simulink model "lab2_part1"  (R2023b)
settings: Solver=VariableStepAuto  StartTime=0.0  StopTime=30.0  RelTol=1e-10  AbsTol=1e-10
undefined symbols (not defined in the file): A, B, K
settings Model: Creator=markzhuang  LastModifiedBy=markzhuang

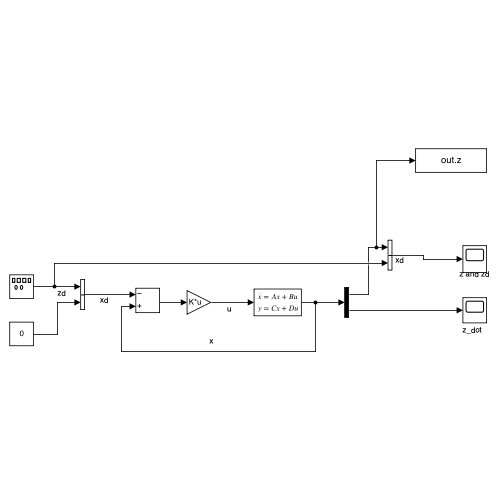
[thumbnail: Simulink's stored preview of the top-level diagram]
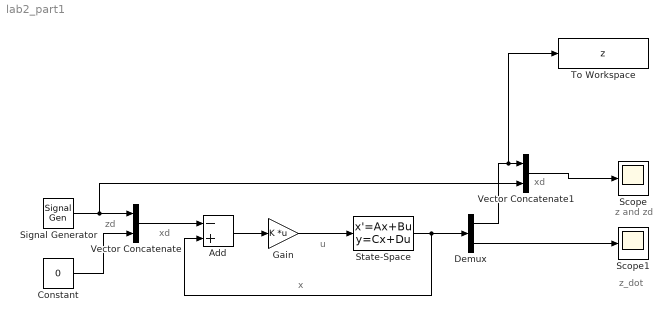
== system lab2_part1 ==
  note: x
  note: u
  note: xd
  note: xd
  note: zd
  note: z_dot
  note: z and zd
  Add : Sum  Inputs=-+
  Constant : Constant  Value=0
  Demux : Demux  Outputs=2
  Gain : Gain  Gain=K  Multiplication=Matrix(K*u)
  Scope : Scope
  Scope1 : Scope
  Signal Generator : SignalGenerator  WaveForm=square  Amplitude=0.03  Frequency=0.1
  State-Space : StateSpace  A=A  B=B  C=[1,0;0,1]  D=[0;0]  InitialCondition=0
  To Workspace : ToWorkspace  VariableName=z  SaveFormat=Timeseries  SampleTime=-1
  Vector Concatenate : Concatenate
  Vector Concatenate1 : Concatenate
  wires:
  Signal Generator/1 -> Vector Concatenate1/2, Vector Concatenate/1
  Constant/1 -> Vector Concatenate/2
  Vector Concatenate/1 -> Add/1
  Demux/2 -> Scope1/1
  Vector Concatenate1/1 -> Scope/1
  Demux/1 -> To Workspace/1, Vector Concatenate1/1
  Add/1 -> Gain/1
  Gain/1 -> State-Space/1
  State-Space/1 -> Add/2, Demux/1
